simulink model "chap02_02_77_mdl"  (R2020a)
settings: Solver=ode45  StartTime=0.0  StopTime=10.0  RelTol=1e-3  EnableMultiTasking=on
settings Model: Creator=Administrator  LastModifiedBy=chen_w3
settings DataIOCC: LimitDataPoints=on  SaveFormat=Array  ReturnWorkspaceOutputs=off
settings OptimizationCC: LifeSpan=inf
settings DebuggingCC: UnderspecifiedInitializationDetection=Classic  MergeDetectMultiDrivingBlocksExec=none  SolverPrmCheckMsg=warning  SFUnexpectedBacktrackingDiag=warning  SFNoUnconditionalDefaultTransitionDiag=warning  SFExecutionAtInitializationDiag=none  ArithmeticOperatorsInVariantConditions=warning
settings HardwareCC: ProdBitPerPointer=32  ProdBitPerSizeT=32  ProdBitPerPtrDiffT=32  ProdLargestAtomicFloat=None  ProdIntDivRoundTo=Undefined  ProdEndianess=Unspecified  ProdWordSize=32  ProdHWDeviceType=32-bit Generic
settings ModelReferenceCC: PropagateSignalLabelsOutOfModel=off
settings SFSimCC: SimUseLocalCustomCode=off  CustomCodeUndefinedFunction=UseInterfaceOnly
settings RTWCC: RTWUseLocalCustomCode=off
settings CodeAppCC: StateflowObjectComments=on
settings GRTTargetCC: TargetLangStandard=C89/C90 (ANSI)
settings ConfigComp: CovMetricSettings=dw  CovHtmlReporting=on  CovSaveCumulativeToWorkspaceVar=on  CovSaveSingleToWorkspaceVar=on  CovExternalEMLEnable=off

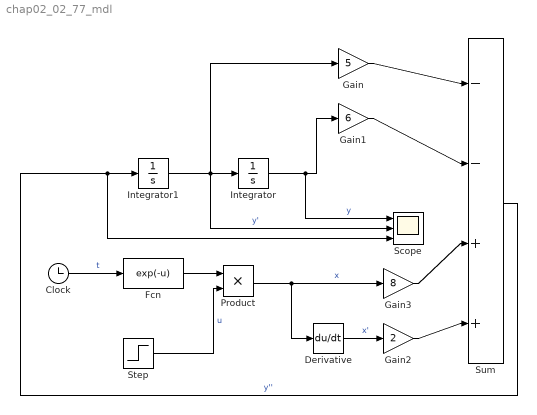
== system chap02_02_77_mdl ==
  Clock : Clock
  Derivative : Derivative
  Fcn : Fcn  Expr=exp(-u)
      mask Display: disp('exp(-t)');
  Gain : Gain  Gain=5
  Gain1 : Gain  Gain=6
  Gain2 : Gain  Gain=2
  Gain3 : Gain  Gain=8
  Integrator : Integrator  InitialCondition=5
      settings: AttributesFormatString=InitVal = %<InitialCondition>
  Integrator1 : Integrator  InitialCondition=-4
      settings: AttributesFormatString=InitVal = %<InitialCondition>
  Product : Product
  Scope : Scope  NumInputPorts=3
  Step : Step  Time=4  SampleTime=0
  Sum : Sum  Inputs=--||++
  wires:
  Integrator1/1 -> Scope/2, Gain/1, Integrator/1  "y'"
  Sum/1 -> Scope/3, Integrator1/1  "y''"
  Integrator/1 -> Scope/1, Gain1/1  "y"
  Clock/1 -> Fcn/1  "t"
  Fcn/1 -> Product/1
  Step/1 -> Product/2  "u"
  Product/1 -> Derivative/1, Gain3/1  "x"
  Derivative/1 -> Gain2/1  "x'"
  Gain2/1 -> Sum/4
  Gain3/1 -> Sum/3
  Gain/1 -> Sum/1
  Gain1/1 -> Sum/2
